simulink model "AHRS"  (R2014b)
settings: Solver=ode8  SolverMode=SingleTasking  StartTime=0.0  StopTime=endtime_selfdefine  FixedStep=0.0025  RelTol=1e-3
InitFcn:
  | %load QuadCopterParameters
values from neighbouring files (symbols this model uses):
  Discretetime_400Hz = 0.0025    [euler_roll_angle_cd.mat]
undefined symbols (not defined in the file or in its folder): dc, g, kalman_gyro, kalman_v
libraries: Lib_AP_AHRS x6, Lib_Sensors x2, Lib_AC_PID x2, simulink x2, Lib_AC_AttitudeControl x1
settings Model: Creator=Ehang  LastModifiedBy=Ehang
settings DataIOCC: SaveOutput=off  SaveTime=off
settings DebuggingCC: SignalInfNanChecking=warning  InheritedTsInSrcMsg=none  UnconnectedInputMsg=none  UnconnectedOutputMsg=none  UnconnectedLineMsg=none
settings ModelReferenceCC: ModelReferenceNumInstancesAllowed=Single
settings GRTTargetCC: MatFileLogging=off

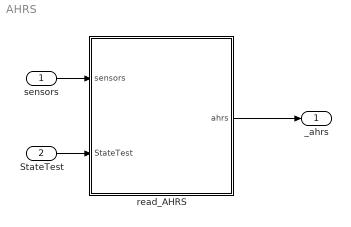
== system AHRS ==
  sensors : Inport  OutDataTypeStr=Bus: Sensors
  StateTest : Inport  Port=2  OutDataTypeStr=Bus: VehicleStates
  read_AHRS : Subsystem
  _ahrs : Outport  OutDataTypeStr=Bus: VehicleStates
  wires:
  sensors/1 -> read_AHRS/1(sensors)
  StateTest/1 -> read_AHRS/2(StateTest)
  read_AHRS/1(ahrs) -> _ahrs/1

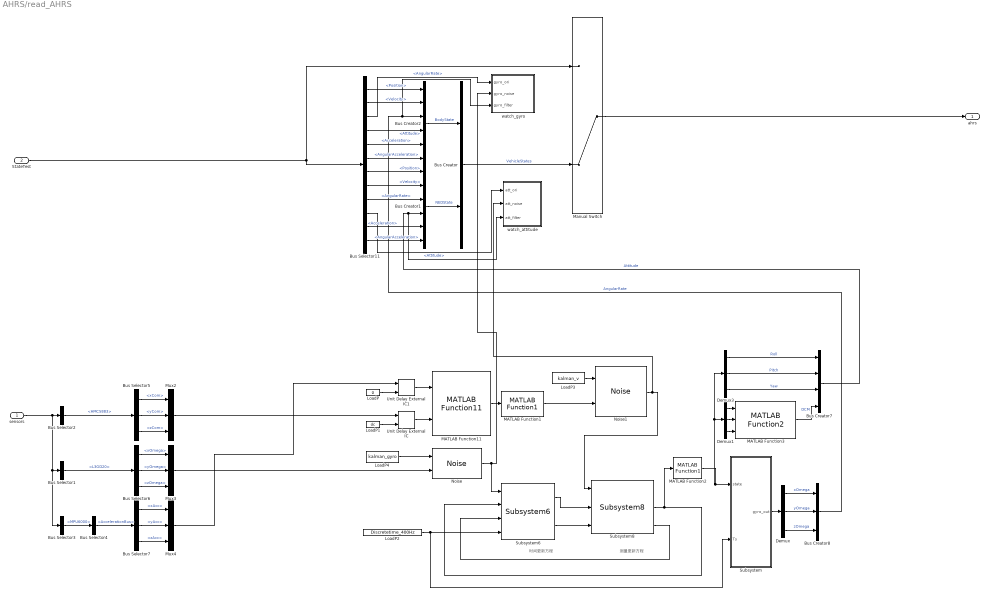
== system AHRS/read_AHRS ==
  note: 时间更新方程
  note: 测量更新方程
  sensors : Inport  OutDataTypeStr=Bus: Sensors
  StateTest : Inport  Port=2  OutDataTypeStr=Bus: VehicleStates
  Bus Creator : BusCreator  Inputs=2  OutDataTypeStr=Bus: VehicleStates
  Bus Creator1 : BusCreator  Inputs=6  OutDataTypeStr=Bus: States
  Bus Creator2 : BusCreator  Inputs=6  OutDataTypeStr=Bus: States
  Bus Creator7 : BusCreator  OutDataTypeStr=Bus: AttitudeBus
  Bus Creator8 : BusCreator  Inputs=3  OutDataTypeStr=Bus: AngularRateBus
  Bus Selector1 : BusSelector  OutputSignals=L3GD20
  Bus Selector11 : BusSelector  OutputSignals=BodyState.Position,BodyState.Velocity,BodyState.AngularRate,BodyState.Attitude,BodyState.Acceleration,BodyState.AngularAcceleration,NEDState.Position,NEDState.Velocity,NEDState.AngularRate,NEDState.Attitude,NEDState.Acceleration,NEDState.AngularAcceleration
  Bus Selector2 : BusSelector  OutputSignals=HMC5883
  Bus Selector3 : BusSelector  OutputSignals=MPU6000
  Bus Selector4 : BusSelector  OutputSignals=AccelerationBus
  Bus Selector5 : BusSelector  OutputSignals=xCom,yCom,zCom
  Bus Selector6 : BusSelector  OutputSignals=xOmega,yOmega,zOmega
  Bus Selector7 : BusSelector  OutputSignals=xAcc,yAcc,zAcc
  Demux : Demux  Outputs=3
  Demux1 : Demux  Outputs=3
  Demux3 : Demux  Outputs=3
  LoadP : Constant  Value=g  SampleTime=0.0025
  LoadP1 : Constant  Value=dc  SampleTime=0.0025
  LoadP2 : Constant  Value=Discretetime_400Hz  SampleTime=-1
  LoadP3 : Constant  Value=kalman_v  SampleTime=0.0025
  LoadP4 : Constant  Value=kalman_gyro  SampleTime=0.0025
  MATLAB Function1 : Lib_AP_AHRS/MATLAB Function1
  MATLAB Function11 : Lib_AP_AHRS/MATLAB Function11
  MATLAB Function2 : Lib_AP_AHRS/MATLAB Function1
  MATLAB Function3 : Lib_AP_AHRS/MATLAB Function2
  Manual Switch : ManualSwitch  CurrentSetting=0
  Mux2 : Mux  Inputs=3
  Mux3 : Mux  Inputs=3
  Mux4 : Mux  Inputs=3
  Noise : Lib_Sensors/Noise
  Noise1 : Lib_Sensors/Noise
  Subsystem : Subsystem
  Subsystem6 : Lib_AP_AHRS/Subsystem6
  Subsystem8 : Lib_AP_AHRS/Subsystem8
  Unit Delay External IC : simulink/Additional Math & Discrete/Additional Discrete/Unit Delay External IC  tsamp=0.0025
  Unit Delay External IC1 : simulink/Additional Math & Discrete/Additional Discrete/Unit Delay External IC  tsamp=0.0025
  watch_attitude : Subsystem
  watch_gyro : Subsystem
  ahrs : Outport
  wires:
  LoadP1/1 -> Unit Delay External IC/2
  LoadP/1 -> Unit Delay External IC1/2
  Mux4/1 -> Unit Delay External IC1/1
  Unit Delay External IC1/1 -> MATLAB Function11/1
  Unit Delay External IC/1 -> MATLAB Function11/2
  MATLAB Function1/1 -> Noise1/2
  Subsystem6/1 -> Subsystem8/2
  Subsystem6/2 -> Subsystem8/3
  Subsystem8/2 -> MATLAB Function2/1, Subsystem6/2
  Subsystem8/3 -> Subsystem6/3
  LoadP2/1 -> Subsystem6/4, Subsystem/2(Ts)
  LoadP3/1 -> Noise1/1
  Noise/1 -> watch_gyro/2(gyro_noise), Subsystem6/1
  LoadP4/1 -> Noise/1
  Subsystem/1(gyro_out) -> Demux/1
  sensors/1 -> Bus Selector3/1, Bus Selector1/1, Bus Selector2/1
  Bus Selector3/1 -> Bus Selector4/1  "<MPU6000>"
  Mux2/1 -> Unit Delay External IC/1
  Mux3/1 -> Noise/2
  Bus Selector1/1 -> Bus Selector6/1  "<L3GD20>"
  Bus Selector2/1 -> Bus Selector5/1  "<HMC5883>"
  Bus Selector4/1 -> Bus Selector7/1  "<AccelerationBus>"
  Bus Selector5/1 -> Mux2/1  "<xCom>"
  Bus Selector5/2 -> Mux2/2  "<yCom>"
  Bus Selector5/3 -> Mux2/3  "<zCom>"
  Bus Selector7/1 -> Mux4/1  "<xAcc>"
  Bus Selector7/2 -> Mux4/2  "<yAcc>"
  Bus Selector7/3 -> Mux4/3  "<zAcc>"
  StateTest/1 -> Bus Selector11/1, Manual Switch/1
  Bus Selector11/2 -> Bus Creator2/2  "<Velocity>"
  Bus Selector11/1 -> Bus Creator2/1  "<Position>"
  Bus Selector11/4 -> Bus Creator2/4  "<Attitude>"
  Bus Selector11/5 -> Bus Creator2/5  "<Acceleration>"
  Bus Selector11/6 -> Bus Creator2/6  "<AngularAcceleration>"
  Bus Selector11/7 -> Bus Creator1/1  "<Position>"
  Bus Selector11/8 -> Bus Creator1/2  "<Velocity>"
  Bus Selector11/9 -> Bus Creator1/3  "<AngularRate>"
  Bus Selector11/11 -> Bus Creator1/5  "<Acceleration>"
  Bus Selector11/12 -> Bus Creator1/6  "<AngularAcceleration>"
  Bus Creator2/1 -> Bus Creator/1  "BodyState"
  Bus Creator1/1 -> Bus Creator/2  "NEDState"
  Bus Creator/1 -> Manual Switch/2  "VehicleStates"
  Bus Selector6/1 -> Mux3/1  "<xOmega>"
  Bus Selector6/2 -> Mux3/2  "<yOmega>"
  Bus Selector6/3 -> Mux3/3  "<zOmega>"
  Demux/1 -> Bus Creator8/1  "xOmega"
  Demux/2 -> Bus Creator8/2  "yOmega"
  Demux/3 -> Bus Creator8/3  "zOmega"
  Bus Creator8/1 -> watch_gyro/3(gyro_filter), Bus Creator2/3  "AngularRate"
  MATLAB Function2/1 -> Subsystem/1(state), Demux3/1, Demux1/1
  MATLAB Function3/1 -> Bus Creator7/4  "DCM"
  Demux3/1 -> Bus Creator7/1  "Roll"
  Demux3/2 -> Bus Creator7/2  "Pitch"
  Bus Creator7/1 -> watch_attitude/3(att_filter), Bus Creator1/4  "Attitude"
  Demux3/3 -> Bus Creator7/3  "Yaw"
  Manual Switch/1 -> ahrs/1
  Demux1/1 -> MATLAB Function3/1
  Demux1/2 -> MATLAB Function3/2
  Demux1/3 -> MATLAB Function3/3
  MATLAB Function11/1 -> MATLAB Function1/1
  Bus Selector11/3 -> watch_gyro/1(gyro_ori)  "<AngularRate>"
  Bus Selector11/10 -> watch_attitude/1(att_ori)  "<Attitude>"
  Noise1/1 -> Subsystem8/1, watch_attitude/2(att_noise)

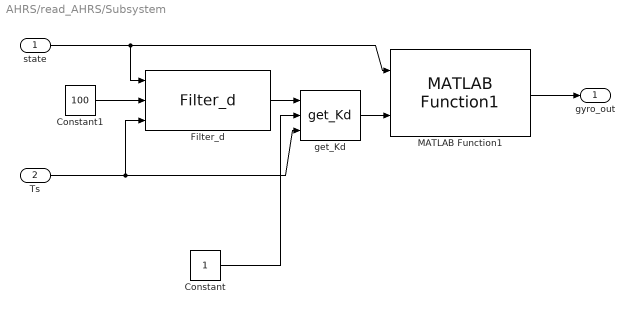
== system AHRS/read_AHRS/Subsystem ==
  state : Inport
  Ts : Inport  Port=2
  Constant : Constant
  Constant1 : Constant  Value=100
  Filter_d : Lib_AC_PID/Filter_d  Description=Tz是时间常数。时间常数一般不小于0.01，否则会振荡。
  MATLAB Function1 : Lib_AC_AttitudeControl/MATLAB Function1
  get_Kd : Lib_AC_PID/get_Kd
  gyro_out : Outport
  wires:
  state/1 -> MATLAB Function1/1, Filter_d/1
  get_Kd/1 -> MATLAB Function1/2
  MATLAB Function1/1 -> gyro_out/1
  Ts/1 -> get_Kd/3, Filter_d/3
  Constant/1 -> get_Kd/2
  Filter_d/1 -> get_Kd/1
  Constant1/1 -> Filter_d/2

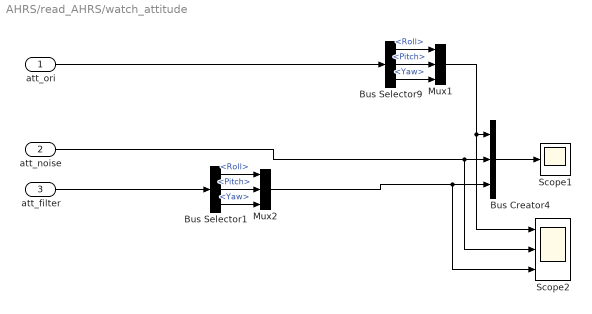
== system AHRS/read_AHRS/watch_attitude ==
  att_ori : Inport  OutDataTypeStr=Bus: AttitudeBus
  att_noise : Inport  Port=2
  att_filter : Inport  Port=3
  Bus Creator4 : BusCreator  Inputs=3
  Bus Selector1 : BusSelector  OutputSignals=Roll,Pitch,Yaw
  Bus Selector9 : BusSelector  OutputSignals=Roll,Pitch,Yaw
  Mux1 : Mux  Inputs=3
  Mux2 : Mux  Inputs=3
  Scope1 : Scope
  Scope2 : Scope  NumInputPorts=3
      settings: YMin=-5~-5~-5  YMax=5~5~5
  wires:
  Mux1/1 -> Scope2/1, Bus Creator4/1
  Bus Selector9/2 -> Mux1/2  "<Pitch>"
  Bus Selector9/1 -> Mux1/1  "<Roll>"
  Bus Selector9/3 -> Mux1/3  "<Yaw>"
  Bus Creator4/1 -> Scope1/1
  att_ori/1 -> Bus Selector9/1
  att_noise/1 -> Scope2/2, Bus Creator4/2
  Bus Selector1/2 -> Mux2/2  "<Pitch>"
  Bus Selector1/1 -> Mux2/1  "<Roll>"
  Bus Selector1/3 -> Mux2/3  "<Yaw>"
  Mux2/1 -> Scope2/3, Bus Creator4/3
  att_filter/1 -> Bus Selector1/1

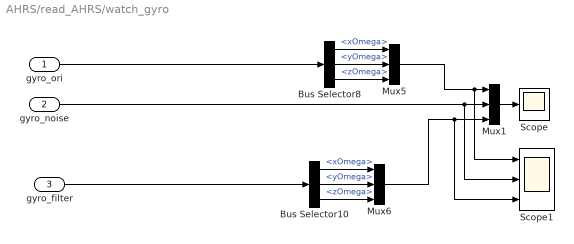
== system AHRS/read_AHRS/watch_gyro ==
  gyro_ori : Inport  OutDataTypeStr=Bus: AngularRateBus
  gyro_noise : Inport  Port=2
  gyro_filter : Inport  Port=3  OutDataTypeStr=Bus: AngularRateBus
  Bus Selector10 : BusSelector  OutputSignals=xOmega,yOmega,zOmega
  Bus Selector8 : BusSelector  OutputSignals=xOmega,yOmega,zOmega
  Mux1 : Mux  Inputs=3
  Mux5 : Mux  Inputs=3
  Mux6 : Mux  Inputs=3
  Scope : Scope
  Scope1 : Scope  NumInputPorts=3
      settings: YMin=-5~-5~-5  YMax=5~5~5
  wires:
  gyro_ori/1 -> Bus Selector8/1
  Bus Selector10/3 -> Mux6/3  "<zOmega>"
  Bus Selector10/2 -> Mux6/2  "<yOmega>"
  Bus Selector10/1 -> Mux6/1  "<xOmega>"
  Mux1/1 -> Scope/1
  Bus Selector8/1 -> Mux5/1  "<xOmega>"
  Bus Selector8/2 -> Mux5/2  "<yOmega>"
  Bus Selector8/3 -> Mux5/3  "<zOmega>"
  Mux5/1 -> Scope1/1, Mux1/1
  gyro_noise/1 -> Scope1/2, Mux1/2
  gyro_filter/1 -> Bus Selector10/1
  Mux6/1 -> Scope1/3, Mux1/3
